simulink model "Handling_2"  (R2025b)
settings: Solver=VariableStepAuto  StartTime=0.0  StopTime=10.0  RelTol=1e-3
libraries: opcualib x1
settings Model: Creator=guilh  LastModifiedBy=guilh

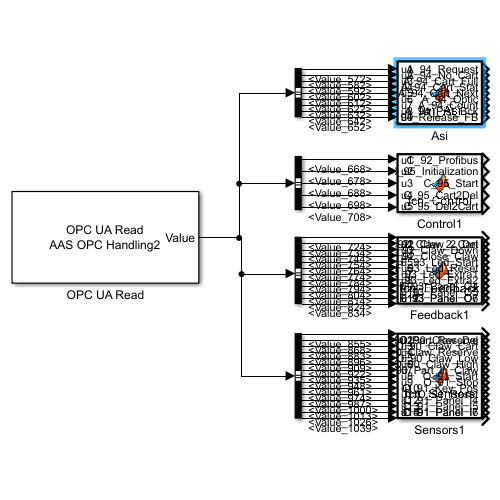
[thumbnail: Simulink's stored preview of the top-level diagram]
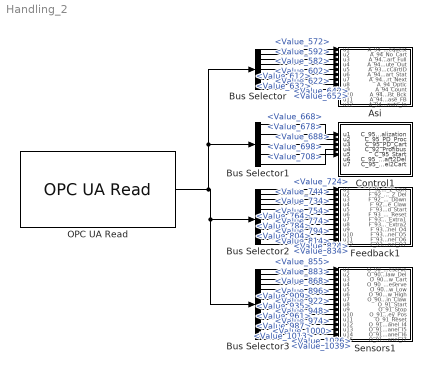
== system Handling_2 ==
  Asi : MATLAB Function  TreatAsAtomicUnit=on
  Bus Selector : BusSelector  OutputSignals=Value_572,Value_582,Value_592,Value_602,Value_612,Value_622,Value_632,Value_642,Value_652
  Bus Selector1 : BusSelector  OutputSignals=Value_668,Value_678,Value_688,Value_698,Value_708
  Bus Selector2 : BusSelector  OutputSignals=Value_724,Value_734,Value_744,Value_754,Value_764,Value_774,Value_784,Value_794,Value_804,Value_814,Value_824,Value_834
  Bus Selector3 : BusSelector  OutputSignals=Value_855,Value_868,Value_883,Value_896,Value_909,Value_922,Value_935,Value_948,Value_961,Value_974,Value_987,Value_1000,Value_1013,Value_1026,Value_1039
  Control1 : MATLAB Function  TreatAsAtomicUnit=on
  Feedback1 : MATLAB Function  TreatAsAtomicUnit=on
  OPC UA Read : opcualib/OPC UA Read  SelectedServer=AAS OPC Handling2  ServerList=AAS OPC Handling2  NodeList={ '1', 'Value', '6', '572', '1'; '2', 'Value', '6', '582', '1'; '3', 'Value', '6', '592', '1'; '4', 'Value', '6', '602', '1'; '5', 'Value', '6', '612', '1'; '6', 'Value', '6', '622', '1'; '7', 'Value', '6', '632', '1'; '8', 'Value', '6', '642', '1'; '9', 'Value', '6', '652', '1'; '10', 'Value', '6', '668', '1'; '11', 'Value', '6', '678', '1'; '12', 'Value', '6', '688', '1'; '13', 'Value', '6', '698', '1'; '14', 'Value', '6', '708', '1'; '15', 'Value', '6', '724', '1'; '16', 'Value', '6', '734', '1'; '17', 'Value', '6', '744', '1'; '18', 'Value', '6', '754', '1'; '19', 'Value', '6', '764', '1'; '20', 'Value', '6', '774', '1'; '21', 'Value', '6', '784', '1'; '22', 'Value', '6', '794', '1'; '23', 'Value', '6', '804', '1'; '24', 'Value', '6', '814', '1'; '25', 'Value', '6', '824', '1'; '26', 'Value', '6', '834', '1'; '27', 'Value', '6', '855', '1'; '28', 'Value', '6', '868', '1'; '29', 'Value', '6', '883', '1'; '30', 'Value', '6', '896', '1'; '31', 'Value', '6', '909', '1'; '32', 'Value', '6', '922', '1'; '33', 'Value', '6', '935', '1'; '34', 'Value', '6', '948', '1'; '35', 'Value', '6', '961', '1'; '36', 'Value', '6', '974', '1'; '37', 'Value', '6', '987', '1'; '38', 'Value', '6', '1000', '1'; '39', 'Value', '6', '1013', '1'; '40', 'Value', '6', '1026', '1'; '41', 'Value', '6', '1039', '1' }  ShowQualityPort=off  ShowTimestampPort=off  ShowTimestampPortAs=Seconds since start  SampleTime=-1
  Sensors1 : MATLAB Function  TreatAsAtomicUnit=on
  wires:
  OPC UA Read/1 -> Bus Selector3/1, Bus Selector2/1, Bus Selector/1, Bus Selector1/1
  Bus Selector/1 -> Asi/1(u1)  "<Value_572>"
  Bus Selector/2 -> Asi/2(u2)  "<Value_582>"
  Bus Selector/3 -> Asi/3(u3)  "<Value_592>"
  Bus Selector/4 -> Asi/4(u4)  "<Value_602>"
  Bus Selector/5 -> Asi/5(u5)  "<Value_612>"
  Bus Selector/6 -> Asi/6(u6)  "<Value_622>"
  Bus Selector/7 -> Asi/7(u7)  "<Value_632>"
  Bus Selector/8 -> Asi/8(u8)  "<Value_642>"
  Bus Selector/9 -> Asi/9(u9)  "<Value_652>"
  Bus Selector1/1 -> Control1/1(u1)  "<Value_668>"
  Bus Selector1/2 -> Control1/2(u2)  "<Value_678>"
  Bus Selector1/3 -> Control1/3(u3)  "<Value_688>"
  Bus Selector1/4 -> Control1/4(u4)  "<Value_698>"
  Bus Selector1/5 -> Control1/5(u5)  "<Value_708>"
  Bus Selector2/1 -> Feedback1/1(u1)  "<Value_724>"
  Bus Selector2/2 -> Feedback1/2(u2)  "<Value_734>"
  Bus Selector2/3 -> Feedback1/3(u3)  "<Value_744>"
  Bus Selector2/4 -> Feedback1/4(u4)  "<Value_754>"
  Bus Selector2/5 -> Feedback1/5(u5)  "<Value_764>"
  Bus Selector2/6 -> Feedback1/6(u6)  "<Value_774>"
  Bus Selector2/7 -> Feedback1/7(u7)  "<Value_784>"
  Bus Selector2/8 -> Feedback1/8(u8)  "<Value_794>"
  Bus Selector2/9 -> Feedback1/9(u9)  "<Value_804>"
  Bus Selector2/10 -> Feedback1/10(u10)  "<Value_814>"
  Bus Selector2/11 -> Feedback1/11(u11)  "<Value_824>"
  Bus Selector2/12 -> Feedback1/12(u12)  "<Value_834>"
  Bus Selector3/1 -> Sensors1/1(u1)  "<Value_855>"
  Bus Selector3/2 -> Sensors1/2(u2)  "<Value_868>"
  Bus Selector3/3 -> Sensors1/3(u3)  "<Value_883>"
  Bus Selector3/4 -> Sensors1/4(u4)  "<Value_896>"
  Bus Selector3/5 -> Sensors1/5(u5)  "<Value_909>"
  Bus Selector3/6 -> Sensors1/6(u6)  "<Value_922>"
  Bus Selector3/7 -> Sensors1/7(u7)  "<Value_935>"
  Bus Selector3/8 -> Sensors1/8(u8)  "<Value_948>"
  Bus Selector3/9 -> Sensors1/9(u9)  "<Value_961>"
  Bus Selector3/10 -> Sensors1/10(u10)  "<Value_974>"
  Bus Selector3/11 -> Sensors1/11(u11)  "<Value_987>"
  Bus Selector3/12 -> Sensors1/12(u12)  "<Value_1000>"
  Bus Selector3/13 -> Sensors1/13(u13)  "<Value_1013>"
  Bus Selector3/14 -> Sensors1/14(u14)  "<Value_1026>"
  Bus Selector3/15 -> Sensors1/15(u15)  "<Value_1039>"

== matlab function Handling_2/Sensors1 ==
  data: u1 input; O_90_Part_Reserve output; u2 input; u3 input; u4 input; u5 input; u6 input; u7 input; u8 input; u9 input; u10 input; u11 input; u12 input; u13 input; u14 input; u15 input; O_90_Claw_Del output; O_90_Claw_Cart output; O_90_Claw_Reserve output; O_90_Claw_Low output; O_90_Claw_High output; O_90_Part_in_Claw output; O_91_Start output; O_91_Stop output; O_91_Key_Pos output; O_91_Reset output; O_91_Panel_I4 output; O_91_Panel_I5 output; O_91_Panel_I6 output; O_91_Panel_I7 output
function [O_90_Part_Reserve,O_90_Claw_Del,O_90_Claw_Cart,...
    O_90_Claw_Reserve,O_90_Claw_Low,O_90_Claw_High,O_90_Part_in_Claw,...
    O_91_Start,O_91_Stop,O_91_Key_Pos,O_91_Reset,O_91_Panel_I4,...
    O_91_Panel_I5,O_91_Panel_I6,O_91_Panel_I7] = fcn_Sensors(u1,u2,u3,u4,...
    u5,u6,u7,u8,u9,u10,u11,u12,u13,u14,u15)

O_90_Part_Reserve = u1;
O_90_Claw_Del = u2;
O_90_Claw_Cart = u3;
O_90_Claw_Reserve = u4;
O_90_Claw_Low = u5;
O_90_Claw_High = u6;
O_90_Part_in_Claw = u7;
O_91_Start = u8;
O_91_Stop = u9;
O_91_Key_Pos = u10;
O_91_Reset = u11;
O_91_Panel_I4 = u12;
O_91_Panel_I5 = u13;
O_91_Panel_I6 = u14;
O_91_Panel_I7 = u15;

== matlab function Handling_2/Asi ==
  data: u1 input; A_94_Request output; u2 input; u3 input; u4 input; u5 input; u6 input; u7 input; u8 input; u9 input; A_94_No_Cart output; A_94_Cart_Full output; A_94_CRoute_Out output; A_93_ProcCartID output; A_94_Cart_Stat output; A_94_Cart_Next output; A_94_Optic output; A_94_Count output; A_94_Pist_Bck output; A_94_Release_FB output; u10 input; u11 input; u12 input; A_94_CRoute_In output
function [A_94_Request,A_94_No_Cart,A_94_Cart_Full,A_94_CRoute_Out,...
A_93_ProcCartID,A_94_Cart_Stat,A_94_Cart_Next,A_94_Optic,A_94_Count,...
A_94_Pist_Bck,A_94_Release_FB,A_94_CRoute_In]...
= fcn_Asi(u1,u2,u3,u4,u5,u6,u7,u8,u9,u10,u11,u12)

A_94_Request = u1;
A_94_No_Cart = u2;
A_94_Cart_Full = u3;
A_94_CRoute_Out = u4;
A_93_ProcCartID = u5;
A_94_Cart_Stat = u6;
A_94_Cart_Next = u7;
A_94_Optic = u8;
A_94_Count = u9;
A_94_Pist_Bck = u10;
A_94_Release_FB = u11;
A_94_CRoute_In = u12;

== matlab function Handling_2/Control1 ==
  data: C_95_Initialization output; C_95_PD_Proc output; C_95_PD_Cart output; u1 input; C_92_Profibus output; u2 input; u3 input; u4 input; u5 input; C_95_Start output; C_95_Cart2Del output; C_95_Del2Cart output; u6 input; u7 input
function [C_95_Initialization,C_95_PD_Proc,C_95_PD_Cart,C_92_Profibus,...
C_95_Start,C_95_Cart2Del,C_95_Del2Cart]...
= fcn_Control(u1,u2,u3,u4,u5,u6,u7)

C_95_Initialization = u1;
C_95_PD_Proc = u2;
C_95_PD_Cart = u3;
C_92_Profibus = u4;
C_95_Start = u5;
C_95_Cart2Del = u6;
C_95_Del2Cart = u7;

== matlab function Handling_2/Feedback1 ==
  data: u1 input; F_92_Claw_2_Cart output; u2 input; u3 input; u4 input; u5 input; u6 input; u7 input; u8 input; u9 input; u10 input; u11 input; u12 input; F_92_Claw_2_Del output; F_92_Claw_Down output; F_92_Close_Claw output; F_93_Led_Start output; F_93_Led_Reset output; F_93_Led_Extra1 output; F_93_Led_Extra2 output; F_93_Panel_O4 output; F_93_Panel_O5 output; F_93_Panel_O6 output; F_93_Panel_O7 output
function [F_92_Claw_2_Cart,F_92_Claw_2_Del,F_92_Claw_Down,...
    F_92_Close_Claw,F_93_Led_Start,F_93_Led_Reset,F_93_Led_Extra1,...
    F_93_Led_Extra2,F_93_Panel_O4,F_93_Panel_O5,F_93_Panel_O6,...
    F_93_Panel_O7] = fcn_Feedback(u1,u2,u3,u4,u5,u6,u7,u8,u9,u10,u11,u12)

F_92_Claw_2_Cart = u1;
F_92_Claw_2_Del = u2;
F_92_Claw_Down = u3;
F_92_Close_Claw = u4;
F_93_Led_Start = u5;
F_93_Led_Reset = u6;
F_93_Led_Extra1 = u7;
F_93_Led_Extra2 = u8;
F_93_Panel_O4 = u9;
F_93_Panel_O5 = u10;
F_93_Panel_O6 = u11;
F_93_Panel_O7 = u12;
